simulink model "Project_Audio"  (R2022a)
settings: Solver=VariableStepAuto  StartTime=0.0  StopTime=15.0  RelTol=1e-3
undefined symbols (not defined in the file): dfilt
libraries: dsparch4 x4, dspvision x3, audioeffects x2, dspsnks4 x1
settings Model: Creator=gouth  LastModifiedBy=gouth

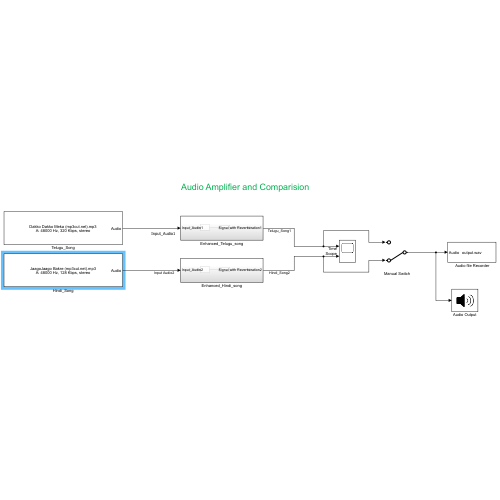
[thumbnail: Simulink's stored preview of the top-level diagram]
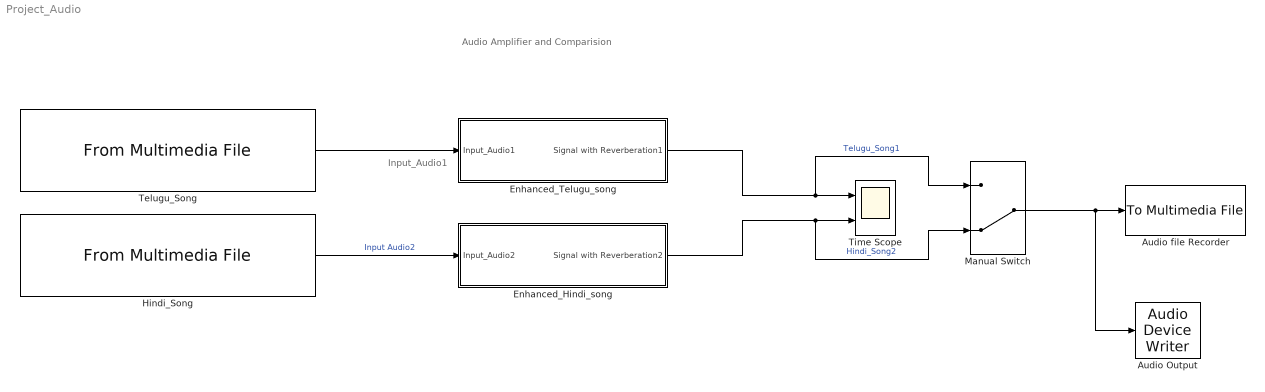
== system Project_Audio ==
  note: Audio Amplifier and Comparision
  note: Input_Audio1
  " Audio file Recorder" : dspvision/To Multimedia File  outputFilename=E:\MathWorks\Project\audio_cut\output.wav  streamSelection=Audio only  videoCompressor=None (uncompressed)  audioCompressor=None (uncompressed)  imagePorts=Separate color signals  fileType=WAV  audioDatatype=16-bit integer  fourcc=RGB  videoQuality=75  mj2000CompFactor=10
  " Manual Switch" : ManualSwitch  CurrentSetting=0
  Audio Output : dspsnks4/Audio Device Writer  Driver=DirectSound  Device=Default  InheritSampleRate=on  SampleRate=44100  BitDepth=16-bit integer  BufferSize=4096  NumBuffers=10  DefaultOutputChannelMapping=on  OutputChannelMapping=1:2  OutputNumUnderrunSamples=off  DriverIdx=1  DeviceWarnFlag=''
  Enhanced_Hindi_song : Subsystem
  Enhanced_Telugu_song : Subsystem
  Hindi_Song : dspvision/From Multimedia File  inputFilename=E:\MathWorks\Project\audio_cut\Puspha\JaagoJaago Bakre (mp3cut.net).mp3  readRange=[1 Inf]  loop=on  numPlays=inf  outputStreams=Audio only  videoDataType=single  audioDataType=double  inheritSampleTime=on  userDefinedSampleTime=1/30  noAudioOutput=off  isIntensityVideo=off  fourcc=RGB  colorVideoFormat=Separate color signals  outputEOF=off  dataOrg=Column-major  audioFrameSize=1026  computeAudioFrameSize=off  outSamplingMode=Sample based
  Telugu_Song : dspvision/From Multimedia File  inputFilename=E:\MathWorks\Project\audio_cut\Puspha\Dakko Dakko Meka (mp3cut.net).mp3  readRange=[1 Inf]  loop=on  numPlays=inf  outputStreams=Audio only  videoDataType=single  audioDataType=double  inheritSampleTime=on  userDefinedSampleTime=1/30  noAudioOutput=off  isIntensityVideo=off  fourcc=RGB  colorVideoFormat=Separate color signals  outputEOF=off  dataOrg=Column-major  audioFrameSize=1026  computeAudioFrameSize=off  outSamplingMode=Sample based
  Time Scope : Scope  NumInputPorts=2
  wires:
  Enhanced_Telugu_song/1(Signal with Reverberation1) -> " Manual Switch"/1, Time Scope/1  "Telugu_Song1"
  Telugu_Song/1 -> Enhanced_Telugu_song/1(Input_Audio1)
  Enhanced_Hindi_song/1(Signal with Reverberation2) -> " Manual Switch"/2, Time Scope/2  "Hindi_Song2"
  Hindi_Song/1 -> Enhanced_Hindi_song/1(Input_Audio2)  "Input Audio2"
  " Manual Switch"/1 -> Audio Output/1, " Audio file Recorder"/1

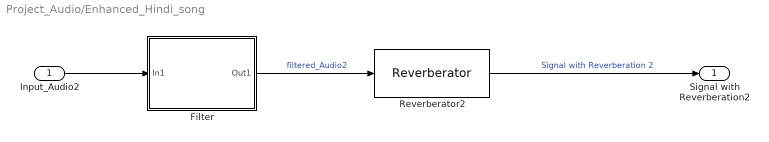
== system Project_Audio/Enhanced_Hindi_song ==
  Input_Audio2 : Inport
  "Filter " : Subsystem
  Reverberator2 : audioeffects/Reverberator  PreDelayPort=off  PreDelay=0.150  HighCutFrequencyPort=off  HighCutFrequency=20000  DiffusionPort=off  Diffusion=0.470  DecayFactorPort=off  DecayFactor=0.330  HighFrequencyDampingPort=off  HighFrequencyDamping=0.270  WetDryMixPort=off  WetDryMix=0.460  InheritSampleRate=on  SampleRate=44100  SimulateUsing=Interpreted execution
      settings: SourceProductBaseCode=AU
  Signal with Reverberation2 : Outport
  wires:
  "Filter "/1(Out1) -> Reverberator2/1  "filtered_Audio2"
  Input_Audio2/1 -> "Filter "/1(In1)
  Reverberator2/1 -> Signal with Reverberation2/1  "Signal with Reverberation 2"

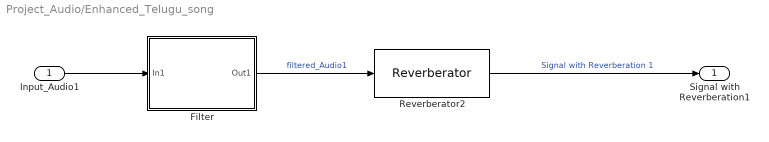
== system Project_Audio/Enhanced_Telugu_song ==
  Input_Audio1 : Inport
  "Filter " : Subsystem
  Reverberator2 : audioeffects/Reverberator  PreDelayPort=off  PreDelay=0.150  HighCutFrequencyPort=off  HighCutFrequency=20000  DiffusionPort=off  Diffusion=0.470  DecayFactorPort=off  DecayFactor=0.330  HighFrequencyDampingPort=off  HighFrequencyDamping=0.270  WetDryMixPort=off  WetDryMix=0.460  InheritSampleRate=on  SampleRate=44100  SimulateUsing=Interpreted execution
      settings: SourceProductBaseCode=AU
  Signal with Reverberation1 : Outport
  wires:
  "Filter "/1(Out1) -> Reverberator2/1  "filtered_Audio1"
  Input_Audio1/1 -> "Filter "/1(In1)
  Reverberator2/1 -> Signal with Reverberation1/1  "Signal with Reverberation 1"

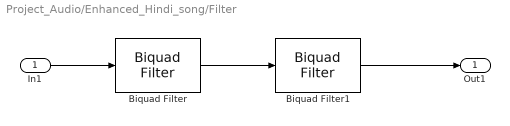
== system Project_Audio/Enhanced_Hindi_song/Filter  ==
  In1 : Inport
  Biquad Filter : dsparch4/Biquad Filter  FilterSource=Dialog parameters  CoeffSource=Specify via dialog  FilterObject=dfilt.df2tsos([1 0.3 0.4],[1 0.1 0.2])  IIRFiltStruct=Direct form II transposed  BiQuadCoeffs=[1 0.3 0.4 1 0.1 0.2]  ScaleValues=1  IC=0  ICnum=0  ICden=0  a0Flag=Warning  optimizeScaleValues=on  ScaleValueMode=Specify via input port (g)  roundingMode=Floor  overflowMode=off  scaleValueFracLength=14  denProdOutputFracLength=30  denAccumFracLength=30  secondMemoryFracLength=15
  Biquad Filter1 : dsparch4/Biquad Filter  FilterSource=Dialog parameters  CoeffSource=Specify via dialog  FilterObject=dfilt.df2tsos([1 0.3 0.4],[1 0.1 0.2])  IIRFiltStruct=Direct form II transposed  BiQuadCoeffs=[1 0.3 0.4 1 0.1 0.2]  ScaleValues=1  IC=0  ICnum=0  ICden=0  a0Flag=Warning  optimizeScaleValues=on  ScaleValueMode=Specify via input port (g)  roundingMode=Floor  overflowMode=off  scaleValueFracLength=14  denProdOutputFracLength=30  denAccumFracLength=30  secondMemoryFracLength=15
  Out1 : Outport
  wires:
  In1/1 -> Biquad Filter/1
  Biquad Filter/1 -> Biquad Filter1/1
  Biquad Filter1/1 -> Out1/1

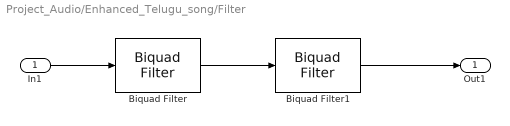
== system Project_Audio/Enhanced_Telugu_song/Filter  ==
  In1 : Inport
  Biquad Filter : dsparch4/Biquad Filter  FilterSource=Dialog parameters  CoeffSource=Specify via dialog  FilterObject=dfilt.df2tsos([1 0.3 0.4],[1 0.1 0.2])  IIRFiltStruct=Direct form II transposed  BiQuadCoeffs=[1 0.3 0.4 1 0.1 0.2]  ScaleValues=1  IC=0  ICnum=0  ICden=0  a0Flag=Warning  optimizeScaleValues=on  ScaleValueMode=Specify via input port (g)  roundingMode=Floor  overflowMode=off  scaleValueFracLength=14  denProdOutputFracLength=30  denAccumFracLength=30  secondMemoryFracLength=15
  Biquad Filter1 : dsparch4/Biquad Filter  FilterSource=Dialog parameters  CoeffSource=Specify via dialog  FilterObject=dfilt.df2tsos([1 0.3 0.4],[1 0.1 0.2])  IIRFiltStruct=Direct form II transposed  BiQuadCoeffs=[1 0.3 0.4 1 0.1 0.2]  ScaleValues=1  IC=0  ICnum=0  ICden=0  a0Flag=Warning  optimizeScaleValues=on  ScaleValueMode=Specify via input port (g)  roundingMode=Floor  overflowMode=off  scaleValueFracLength=14  denProdOutputFracLength=30  denAccumFracLength=30  secondMemoryFracLength=15
  Out1 : Outport
  wires:
  In1/1 -> Biquad Filter/1
  Biquad Filter/1 -> Biquad Filter1/1
  Biquad Filter1/1 -> Out1/1
